simulink model "io183_voltage_loopback"  (R2026a)
settings: Solver=FixedStepDiscrete  StopTime=inf  FixedStep=0.001
undefined symbols (not defined in the file or in its folder): Pull, up
libraries: speedgoatlib_IO183 x3
settings Model: Creator=aniru  LastModifiedBy=aniru
settings SolverCC: ConcurrentTasks=on  PositivePriorityOrder=on
settings OptimizationCC: OptimizeBlockIOStorage=off
settings DebuggingCC: TasksWithSamePriorityMsg=none
settings HardwareCC: ProdBitPerLong=64.0  ProdHWDeviceType=Intel->x86-64 (Linux 64)
settings RTWCC: SystemTargetFile=speedgoat.tlc  TemplateMakefile=slrealtime_default_tmf  Toolchain=Simulink Real-Time Toolchain  BuildConfiguration=Faster Runs  TargetLang=C++  Description=Speedgoat Real-Time Target Machine
settings SimulinkRealTimeTargetCC: SLRTFileLogMaxRuns=1.0  TargetLangStandard=C++11 (ISO)  MultiwordLength=2048.0  MATLABClassNameForMDSCustomization=Simulink.SoftwareTarget.GRTCustomization

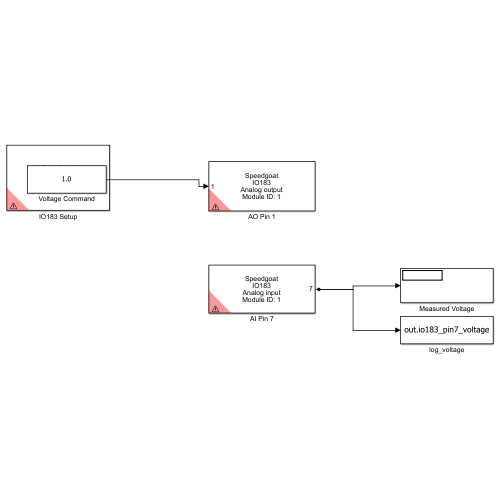
[thumbnail: Simulink's stored preview of the top-level diagram]
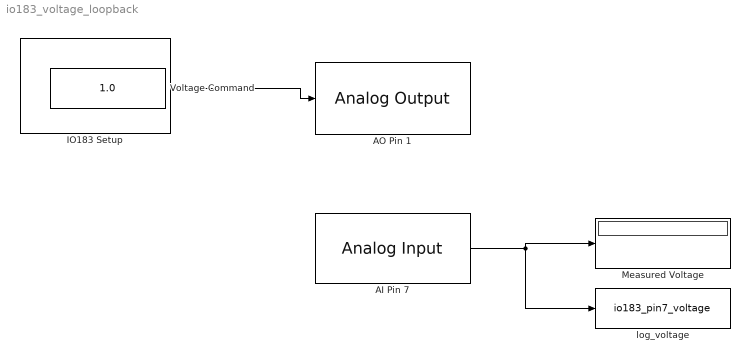
== system io183_voltage_loopback ==
  AI Pin 7 : speedgoatlib_IO183/Analog Input  Priority=0  parModuleId=1  parSampTime=0.001  parPciSlot=-1  parAdChannelLow=7  parAdChannelHigh=7
      settings: SourceProductName=IO183
  AO Pin 1 : speedgoatlib_IO183/Analog Output  parModuleId=1  parSampTime=0.001  parDaSimult=on  parPciSlot=-1  parDaChannels=1  parDaInit=[0 0 0 0]  parDaReset=[0 0 0 0]
      settings: SourceProductName=IO183
  IO183 Setup : speedgoatlib_IO183/Setup  parModuleId=1  parPciSlot=-1  parDaSimult=on  parAdCoupling=Single Ended  parAdRange=+-5V  parAdChannelLow=7  parAdChannelHigh=7  parDaChannels=1  parDaRange=0..5V  parDaInit=0  parDaReset=0  parDoChannels=[1:8]  parDoInit=[0]  parDoReset=[1]  parDiChannels=[9:16]  parIOPullReferenceFront=Pull-up (3.3V)  parIOPullReferenceRear=Pull-up (3.3V)
      settings: SourceProductName=IO183
  Measured Voltage : Display
  Voltage Command : Constant  Value=1.0  SampleTime=0.001
  log_voltage : ToWorkspace  VariableName=io183_pin7_voltage  SaveFormat=Timeseries  SampleTime=-1
  wires:
  Voltage Command/1 -> AO Pin 1/1
  AI Pin 7/1 -> Measured Voltage/1, log_voltage/1
